simulink library "Suspension_Utilities"  (R2024b)
settings: Solver=VariableStepAuto  StartTime=0.0  StopTime=10.0  RelTol=1e-3
undefined symbols (not defined in the file or in its folder): Ac, Af, Ar, hp1, hp2, hp3, hp_in, hp_in_f_ua, hp_in_r_ua, hp_mount_subframe, hp_shk_frame, hp_spr_bot, hp_spr_top, hpb, hpf, hpo, hpx, hpz, Newton, Raphson, rotYAxis, SubframeConnection, Upper_Arm_to_Subframe, Visual, X, Y, Z
libraries: sm_lib x75, $bdroot x23, linkage_bushing_6DOF_lib x13, fl_lib x4, sharedtransformsys x3, linkage_bushing_5DOF_lib x2, nesl_utility x1
(part 4 of 4)

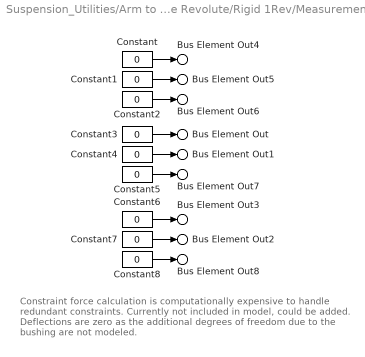
== system Suspension_Utilities/Arm to Subframe Revolute/Rigid 1Rev/Measurements Af ==
  note: Constraint force calculation is computationally expensive to handle redundant constraints.  Currently not included in model, could be added.
      |
      | Deflections are zero as the additional degrees of freedom due to the bushing are not modeled.
  Constant{,1..8} (9 alike) : Constant  Value=0
  Bus Element Out : Outport  PortName=m  Element=vy
  Bus Element Out1 : Outport  PortName=m  Element=py
  Bus Element Out2 : Outport  PortName=m  Element=pz
  Bus Element Out3 : Outport  PortName=m  Element=vz
  Bus Element Out4 : Outport  PortName=m  Element=vx
  Bus Element Out5 : Outport  PortName=m  Element=px
  Bus Element Out6 : Outport  PortName=m  Element=fx
  Bus Element Out7 : Outport  PortName=m  Element=fy
  Bus Element Out8 : Outport  PortName=m  Element=fz
  wires:
  Constant/1 -> Bus Element Out4/1
  Constant2/1 -> Bus Element Out6/1
  Constant1/1 -> Bus Element Out5/1
  Constant4/1 -> Bus Element Out1/1
  Constant5/1 -> Bus Element Out7/1
  Constant3/1 -> Bus Element Out/1
  Constant6/1 -> Bus Element Out3/1
  Constant8/1 -> Bus Element Out8/1
  Constant7/1 -> Bus Element Out2/1

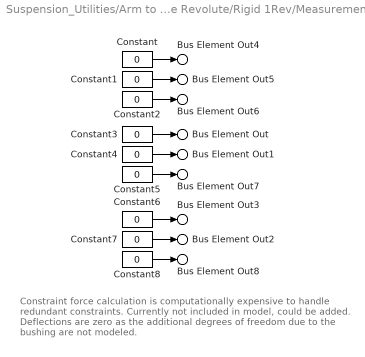
== system Suspension_Utilities/Arm to Subframe Revolute/Rigid 1Rev/Measurements Ar ==
  note: Constraint force calculation is computationally expensive to handle redundant constraints.  Currently not included in model, could be added.
      |
      | Deflections are zero as the additional degrees of freedom due to the bushing are not modeled.
  Constant{,1..8} (9 alike) : Constant  Value=0
  Bus Element Out : Outport  PortName=m  Element=vy
  Bus Element Out1 : Outport  PortName=m  Element=py
  Bus Element Out2 : Outport  PortName=m  Element=pz
  Bus Element Out3 : Outport  PortName=m  Element=vz
  Bus Element Out4 : Outport  PortName=m  Element=vx
  Bus Element Out5 : Outport  PortName=m  Element=px
  Bus Element Out6 : Outport  PortName=m  Element=fx
  Bus Element Out7 : Outport  PortName=m  Element=fy
  Bus Element Out8 : Outport  PortName=m  Element=fz
  wires:
  Constant7/1 -> Bus Element Out2/1
  Constant8/1 -> Bus Element Out8/1
  Constant6/1 -> Bus Element Out3/1
  Constant3/1 -> Bus Element Out/1
  Constant5/1 -> Bus Element Out7/1
  Constant4/1 -> Bus Element Out1/1
  Constant1/1 -> Bus Element Out5/1
  Constant2/1 -> Bus Element Out6/1
  Constant/1 -> Bus Element Out4/1

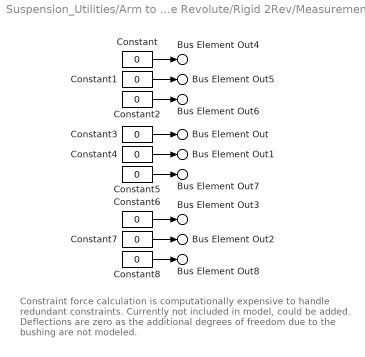
== system Suspension_Utilities/Arm to Subframe Revolute/Rigid 2Rev/Measurements Af ==
  note: Constraint force calculation is computationally expensive to handle redundant constraints.  Currently not included in model, could be added.
      |
      | Deflections are zero as the additional degrees of freedom due to the bushing are not modeled.
  Constant{,1..8} (9 alike) : Constant  Value=0
  Bus Element Out : Outport  PortName=m  Element=vy
  Bus Element Out1 : Outport  PortName=m  Element=py
  Bus Element Out2 : Outport  PortName=m  Element=pz
  Bus Element Out3 : Outport  PortName=m  Element=vz
  Bus Element Out4 : Outport  PortName=m  Element=vx
  Bus Element Out5 : Outport  PortName=m  Element=px
  Bus Element Out6 : Outport  PortName=m  Element=fx
  Bus Element Out7 : Outport  PortName=m  Element=fy
  Bus Element Out8 : Outport  PortName=m  Element=fz
  wires:
  Constant/1 -> Bus Element Out4/1
  Constant2/1 -> Bus Element Out6/1
  Constant1/1 -> Bus Element Out5/1
  Constant4/1 -> Bus Element Out1/1
  Constant5/1 -> Bus Element Out7/1
  Constant3/1 -> Bus Element Out/1
  Constant6/1 -> Bus Element Out3/1
  Constant8/1 -> Bus Element Out8/1
  Constant7/1 -> Bus Element Out2/1

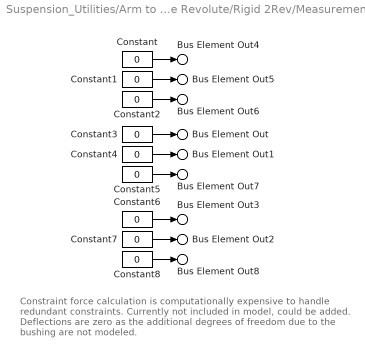
== system Suspension_Utilities/Arm to Subframe Revolute/Rigid 2Rev/Measurements Ar ==
  note: Constraint force calculation is computationally expensive to handle redundant constraints.  Currently not included in model, could be added.
      |
      | Deflections are zero as the additional degrees of freedom due to the bushing are not modeled.
  Constant{,1..8} (9 alike) : Constant  Value=0
  Bus Element Out : Outport  PortName=m  Element=vy
  Bus Element Out1 : Outport  PortName=m  Element=py
  Bus Element Out2 : Outport  PortName=m  Element=pz
  Bus Element Out3 : Outport  PortName=m  Element=vz
  Bus Element Out4 : Outport  PortName=m  Element=vx
  Bus Element Out5 : Outport  PortName=m  Element=px
  Bus Element Out6 : Outport  PortName=m  Element=fx
  Bus Element Out7 : Outport  PortName=m  Element=fy
  Bus Element Out8 : Outport  PortName=m  Element=fz
  wires:
  Constant7/1 -> Bus Element Out2/1
  Constant8/1 -> Bus Element Out8/1
  Constant6/1 -> Bus Element Out3/1
  Constant3/1 -> Bus Element Out/1
  Constant5/1 -> Bus Element Out7/1
  Constant4/1 -> Bus Element Out1/1
  Constant1/1 -> Bus Element Out5/1
  Constant2/1 -> Bus Element Out6/1
  Constant/1 -> Bus Element Out4/1

== system Suspension_Utilities/Arm to Subframe Universal/Rigid UJ/Measurements ==
  note: Constraint force calculation is computationally expensive to handle redundant constraints.  Currently not included in model, could be added.
      |
      | Deflections are zero as the additional degrees of freedom due to the bushing are not modeled.
  Constant{,1..6} (7 alike) : Constant  Value=0
  Bus Element Out : Outport  PortName=m  Element=pr
  Bus Element Out1 : Outport  PortName=m  Element=vr
  Bus Element Out2 : Outport  PortName=m  Element=pa
  Bus Element Out3 : Outport  PortName=m  Element=va
  Bus Element Out4 : Outport  PortName=m  Element=fx
  Bus Element Out5 : Outport  PortName=m  Element=fy
  Bus Element Out6 : Outport  PortName=m  Element=fz
  wires:
  Constant2/1 -> Bus Element Out4/1
  Constant5/1 -> Bus Element Out2/1
  Constant4/1 -> Bus Element Out3/1
  Constant3/1 -> Bus Element Out5/1
  Constant6/1 -> Bus Element Out6/1
  Constant1/1 -> Bus Element Out1/1
  Constant/1 -> Bus Element Out/1

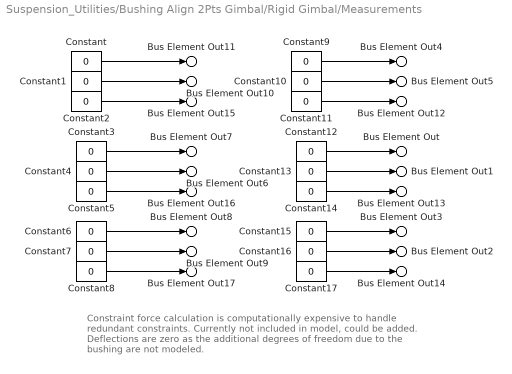
== system Suspension_Utilities/Bushing Align 2Pts Gimbal/Rigid Gimbal/Measurements ==
  note: Constraint force calculation is computationally expensive to handle redundant constraints.  Currently not included in model, could be added.
      |
      | Deflections are zero as the additional degrees of freedom due to the bushing are not modeled.
  Constant{,1..17} (18 alike) : Constant  Value=0
  Bus Element Out : Outport  PortName=m  Element=vy
  Bus Element Out1 : Outport  PortName=m  Element=py
  Bus Element Out2 : Outport  PortName=m  Element=pz
  Bus Element Out3 : Outport  PortName=m  Element=vz
  Bus Element Out4 : Outport  PortName=m  Element=vx
  Bus Element Out5 : Outport  PortName=m  Element=px
  Bus Element Out6 : Outport  PortName=m  Element=qy
  Bus Element Out7 : Outport  PortName=m  Element=wy
  Bus Element Out8 : Outport  PortName=m  Element=wz
  Bus Element Out9 : Outport  PortName=m  Element=qz
  Bus Element Out10 : Outport  PortName=m  Element=qx
  Bus Element Out11 : Outport  PortName=m  Element=wx
  Bus Element Out12 : Outport  PortName=m  Element=fx
  Bus Element Out13 : Outport  PortName=m  Element=fy
  Bus Element Out14 : Outport  PortName=m  Element=fz
  Bus Element Out15 : Outport  PortName=m  Element=tx
  Bus Element Out16 : Outport  PortName=m  Element=ty
  Bus Element Out17 : Outport  PortName=m  Element=tz
  wires:
  Constant/1 -> Bus Element Out11/1
  Constant1/1 -> Bus Element Out10/1
  Constant2/1 -> Bus Element Out15/1
  Constant5/1 -> Bus Element Out16/1
  Constant4/1 -> Bus Element Out6/1
  Constant3/1 -> Bus Element Out7/1
  Constant8/1 -> Bus Element Out17/1
  Constant7/1 -> Bus Element Out9/1
  Constant6/1 -> Bus Element Out8/1
  Constant15/1 -> Bus Element Out3/1
  Constant16/1 -> Bus Element Out2/1
  Constant17/1 -> Bus Element Out14/1
  Constant12/1 -> Bus Element Out/1
  Constant13/1 -> Bus Element Out1/1
  Constant14/1 -> Bus Element Out13/1
  Constant11/1 -> Bus Element Out12/1
  Constant10/1 -> Bus Element Out5/1
  Constant9/1 -> Bus Element Out4/1

== system Suspension_Utilities/Q to Z-Y-X Extrinsic/Subsystem/Subsystem ==
  In : Inport
  If : If  IfExpression=u1 > 1  ElseIfExpressions=u1 < -1
  If Action Subsystem : sharedtransformsys/Protect asincos input/If Action Subsystem  SystemSampleTime=-1  VariantActivationTime=update diagram  Latency=0  AutoFrameSizeCalculation=off
  If Action Subsystem1 : sharedtransformsys/Protect asincos input/If Action Subsystem1  SystemSampleTime=-1  VariantActivationTime=update diagram  Latency=0  AutoFrameSizeCalculation=off
  If Action Subsystem2 : sharedtransformsys/Protect asincos input/If Action Subsystem2  SystemSampleTime=-1  VariantActivationTime=update diagram  Latency=0  AutoFrameSizeCalculation=off
  Merge : Merge  Inputs=3
  Out : Outport  VectorParamsAs1DForOutWhenUnconnected=off
  wires:
  Merge/1 -> Out/1
  If Action Subsystem/1 -> Merge/1
  If/2 -> If Action Subsystem1/Action
  If Action Subsystem2/1 -> Merge/3
  If/3 -> If Action Subsystem2/Action
  In/1 -> If Action Subsystem2/1, If/1
  If/1 -> If Action Subsystem/Action
  If Action Subsystem1/1 -> Merge/2

== system Suspension_Utilities/Q to Z-Y-X Extrinsic/Subsystem1/Subsystem ==
  In1 : Inport
  Demux : Demux
  Product{,1..3} (4 alike) : Product
  Sum : Sum  Inputs=4
  sqrt : Sqrt  AlgorithmType=Newton-Raphson
  Out1 : Outport  VectorParamsAs1DForOutWhenUnconnected=off
  wires:
  Demux/4 -> Product3/2, Product3/1
  Product1/1 -> Sum/2
  Demux/3 -> Product2/2, Product2/1
  Product/1 -> Sum/1
  Product2/1 -> Sum/3
  Demux/1 -> Product/2, Product/1
  Demux/2 -> Product1/2, Product1/1
  Product3/1 -> Sum/4
  In1/1 -> Demux/1
  sqrt/1 -> Out1/1
  Sum/1 -> sqrt/1

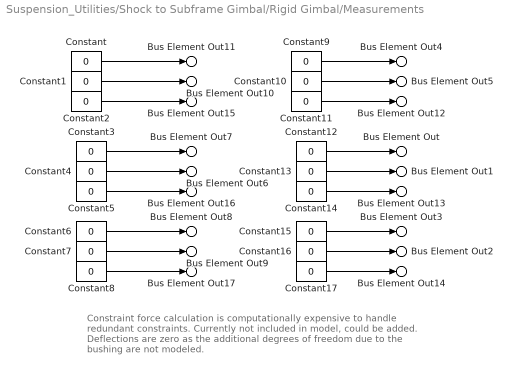
== system Suspension_Utilities/Shock to Subframe Gimbal/Rigid Gimbal/Measurements ==
  note: Constraint force calculation is computationally expensive to handle redundant constraints.  Currently not included in model, could be added.
      |
      | Deflections are zero as the additional degrees of freedom due to the bushing are not modeled.
  Constant{,1..17} (18 alike) : Constant  Value=0
  Bus Element Out : Outport  PortName=m  Element=vy
  Bus Element Out1 : Outport  PortName=m  Element=py
  Bus Element Out2 : Outport  PortName=m  Element=pz
  Bus Element Out3 : Outport  PortName=m  Element=vz
  Bus Element Out4 : Outport  PortName=m  Element=vx
  Bus Element Out5 : Outport  PortName=m  Element=px
  Bus Element Out6 : Outport  PortName=m  Element=qy
  Bus Element Out7 : Outport  PortName=m  Element=wy
  Bus Element Out8 : Outport  PortName=m  Element=wz
  Bus Element Out9 : Outport  PortName=m  Element=qz
  Bus Element Out10 : Outport  PortName=m  Element=qx
  Bus Element Out11 : Outport  PortName=m  Element=wx
  Bus Element Out12 : Outport  PortName=m  Element=fx
  Bus Element Out13 : Outport  PortName=m  Element=fy
  Bus Element Out14 : Outport  PortName=m  Element=fz
  Bus Element Out15 : Outport  PortName=m  Element=tx
  Bus Element Out16 : Outport  PortName=m  Element=ty
  Bus Element Out17 : Outport  PortName=m  Element=tz
  wires:
  Constant/1 -> Bus Element Out11/1
  Constant1/1 -> Bus Element Out10/1
  Constant2/1 -> Bus Element Out15/1
  Constant5/1 -> Bus Element Out16/1
  Constant4/1 -> Bus Element Out6/1
  Constant3/1 -> Bus Element Out7/1
  Constant8/1 -> Bus Element Out17/1
  Constant7/1 -> Bus Element Out9/1
  Constant6/1 -> Bus Element Out8/1
  Constant15/1 -> Bus Element Out3/1
  Constant16/1 -> Bus Element Out2/1
  Constant17/1 -> Bus Element Out14/1
  Constant12/1 -> Bus Element Out/1
  Constant13/1 -> Bus Element Out1/1
  Constant14/1 -> Bus Element Out13/1
  Constant11/1 -> Bus Element Out12/1
  Constant10/1 -> Bus Element Out5/1
  Constant9/1 -> Bus Element Out4/1
